simulink model "Automatisierung_Kapitel8_zustandsbeobachter"  (R2015b)
settings: Solver=ode45  StartTime=0.0  StopTime=100  MaxStep=0.2  RelTol=1e-3
values from neighbouring files (symbols this model uses):
  Ac = [0,1,0,0;-1,-1,1,1;0,0,0,1;0.1,0.1,-0.2,-0.2]    [Automatisierung_Kapitel8.m]
  AdL = Ad+kbeo'*cc    [Automatisierung_Kapitel8.m]
  AdT = Ad    [Automatisierung_Kapitel8.m]
  Bc = [bc,bvc]    [Automatisierung_Kapitel8.m]
  BdL = [bd,-kbeo']    [Automatisierung_Kapitel8.m]
  bdT = bd    [Automatisierung_Kapitel8.m]
  Cc = eye(4)    [Automatisierung_Kapitel8.m]
  CdL = eye(4)    [Automatisierung_Kapitel8.m]
  CdT = eye(4)    [Automatisierung_Kapitel8.m]
  Dc = [0,0;0,0;0,0;0,0]    [Automatisierung_Kapitel8.m]
  DdL = [0,0;0,0;0,0;0,0]    [Automatisierung_Kapitel8.m]
  ddT = [0,0,0,0]'    [Automatisierung_Kapitel8.m]
  Ta = 2    [Automatisierung_Kapitel8.m]
  x0 = [10,0,0,0]    [Automatisierung_Kapitel8.m]
settings Model: Creator=aku  LastModifiedBy=hk
settings DataIOCC: SaveFormat=Array  SignalLoggingSaveFormat=ModelDataLogs
settings OptimizationCC: BooleanDataType=off  ExpressionDepthLimit=2147483647  InitFltsAndDblsToZero=on
settings DebuggingCC: SaveWithParameterizedLinksMsg=none  UnderspecifiedInitializationDetection=Classic  MergeDetectMultiDrivingBlocksExec=none  SignalResolutionControl=TryResolveAllWithWarning  MultiTaskDSMMsg=warning  MultiTaskCondExecSysMsg=none  FcnCallInpInsideContextMsg=EnableAllAsWarning  StateNameClashWarn=warning
settings HardwareCC: ProdBitPerPointer=32  ProdLargestAtomicFloat=None  ProdIntDivRoundTo=Undefined  ProdEndianess=Unspecified  ProdWordSize=32  ProdHWDeviceType=32-bit Generic  TargetUnknown=on
settings GRTTargetCC: TargetFcnLib=ansi_tfl_tmw.mat  GeneratePreprocessorConditionals=Disable all  CombineOutputUpdateFcns=off  GRTInterface=on
settings ConfigComp: CovModelRefEnable=Off  CovSFcnEnable=off

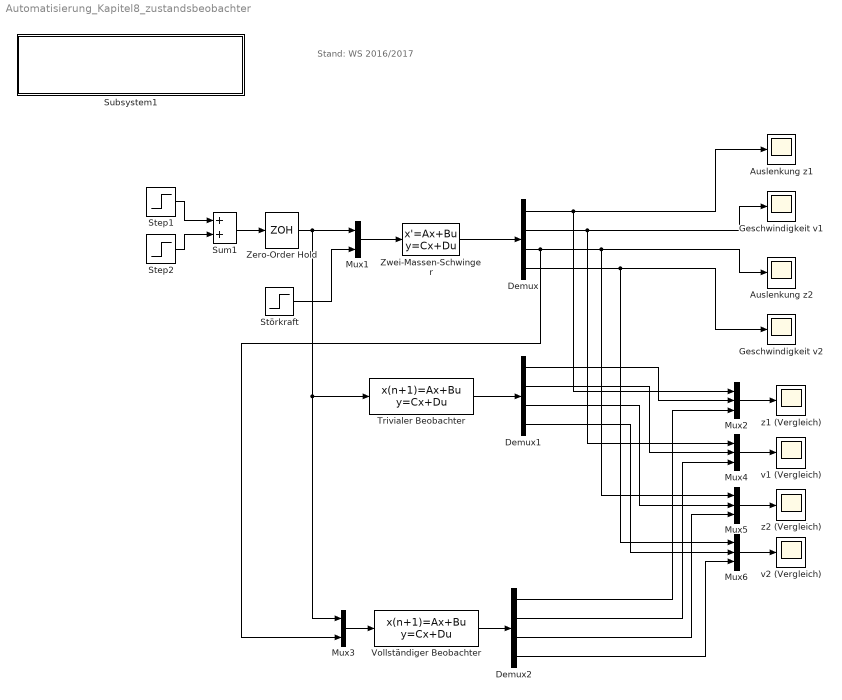
== system Automatisierung_Kapitel8_zustandsbeobachter ==
  note: Stand: WS 2016/2017
  Auslenkung z1 : Scope
  Auslenkung z2 : Scope
  Demux : Demux
  Demux1 : Demux
  Demux2 : Demux
  Geschwindigkeit v1 : Scope
  Geschwindigkeit v2 : Scope
  Mux1 : Mux  Inputs=2
  Mux{2,4..6} (4 alike) : Mux  Inputs=3
  Mux3 : Mux  Inputs=2
  Step1 : Step  Time=0  SampleTime=0
  Step2 : Step  Time=50  After=-2  SampleTime=0
  Störkraft : Step  Time=60  After=0  SampleTime=0
  Subsystem1 : Subsystem
      settings: OpenFcn=Automatisierung_Kapitel8
      mask Display:
      | disp('Daten laden (Automatisierung_Kapitel8.m)\n\n');
      | disp('(mittels Doppelklick)');
  Sum1 : Sum
  Trivialer Beobachter : DiscreteStateSpace  A=AdT  B=bdT  C=CdT  D=ddT  X0=[0,0,0,0]  SampleTime=Ta
  Vollständiger Beobachter : DiscreteStateSpace  A=AdL  B=BdL  C=CdL  D=DdL  X0=[0,0,0,0]  SampleTime=Ta
  Zero-Order Hold : ZeroOrderHold  SampleTime=Ta
  Zwei-Massen-Schwinger : StateSpace  A=Ac  B=Bc  C=Cc  D=Dc  X0=x0
  v1 (Vergleich) : Scope
  v2 (Vergleich) : Scope
  "z1 (Vergleich) " : Scope
  z2 (Vergleich) : Scope
  wires:
  Zwei-Massen-Schwinger/1 -> Demux/1
  Mux1/1 -> Zwei-Massen-Schwinger/1
  Zero-Order Hold/1 -> Mux1/1, Trivialer Beobachter/1, Mux3/1
  Störkraft/1 -> Mux1/2
  Demux/1 -> Auslenkung z1/1, Mux2/1
  Demux/3 -> Auslenkung z2/1, Mux5/1, Mux3/2
  Demux/2 -> Geschwindigkeit v1/1, Mux4/1
  Demux/4 -> Geschwindigkeit v2/1, Mux6/1
  Trivialer Beobachter/1 -> Demux1/1
  Demux1/1 -> Mux2/2
  Demux1/2 -> Mux4/2
  Demux1/3 -> Mux5/2
  Demux1/4 -> Mux6/2
  Mux2/1 -> "z1 (Vergleich) "/1
  Mux4/1 -> v1 (Vergleich)/1
  Mux5/1 -> z2 (Vergleich)/1
  Mux6/1 -> v2 (Vergleich)/1
  Sum1/1 -> Zero-Order Hold/1
  Step1/1 -> Sum1/1
  Step2/1 -> Sum1/2
  Mux3/1 -> Vollständiger Beobachter/1
  Vollständiger Beobachter/1 -> Demux2/1
  Demux2/1 -> Mux2/3
  Demux2/2 -> Mux4/3
  Demux2/3 -> Mux5/3
  Demux2/4 -> Mux6/3

== system Automatisierung_Kapitel8_zustandsbeobachter/Subsystem1 ==
